simulink model "astrobee"  (R2016b)
settings: configuration reference "cset" (kept outside this file)
PreLoadFcn:
  | astrobee_init;
  | astrobee_prep;
values from neighbouring files (symbols this model uses):
  bus_cmc_msg_ic = Simulink.Bus.createMATLABStruct('cmc_msg')    [bus_init.m]
undefined symbols (not defined in the file or in its folder): ase_local_mode_docking, att_ki, att_kp, center_of_mass, inertia_matrix, mass, mlp_loc_mode_cmd_list, mlp_loc_mode_cmd_times, omega_kd, pos_ki, pos_kp, tun_default_att_ki, tun_default_att_kp, tun_default_center_of_mass, tun_default_inertia_matrix, tun_default_mass, tun_default_omega_kd, tun_default_pos_ki, tun_default_pos_kp, tun_default_vel_kd, vel_kd
libraries: simulink x1, cmc_command_and_mode_control x1, fsw_lib x1, sim_model_lib x1
settings Model: Creator=mjmcinty  LastModifiedBy=jfusco1
settings ConfigSetRef: SourceLocation=Base Workspace

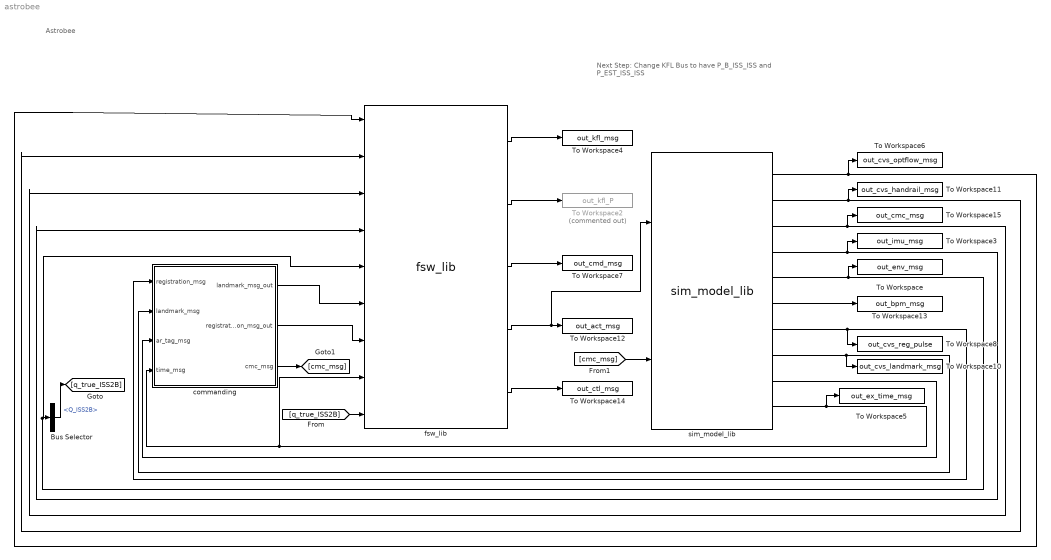
== system astrobee ==
  note: Next Step:
      | Change KFL Bus to have P_B_ISS_ISS and P_EST_ISS_ISS
  note: Astrobee
  Bus Selector : BusSelector  OutputSignals=Q_ISS2B
  To Workspace : ToWorkspace  VariableName=out_env_msg  SaveFormat=Timeseries  SampleTime=-1
  To Workspace10 : ToWorkspace  VariableName=out_cvs_landmark_msg  SaveFormat=Timeseries  SampleTime=-1
  To Workspace11 : ToWorkspace  VariableName=out_cvs_handrail_msg  SaveFormat=Timeseries  SampleTime=-1
  To Workspace12 : ToWorkspace  VariableName=out_act_msg  SaveFormat=Timeseries  SampleTime=-1
  To Workspace13 : ToWorkspace  VariableName=out_bpm_msg  SaveFormat=Timeseries  SampleTime=-1
  To Workspace14 : ToWorkspace  VariableName=out_ctl_msg  SaveFormat=Timeseries  SampleTime=-1
  To Workspace15 : ToWorkspace  VariableName=out_cmc_msg  SaveFormat=Timeseries  SampleTime=-1
  To Workspace2 : ToWorkspace  Commented=on  VariableName=out_kfl_P  SaveFormat=Timeseries  SampleTime=-1
  To Workspace3 : ToWorkspace  VariableName=out_imu_msg  SaveFormat=Timeseries  SampleTime=-1
  To Workspace4 : ToWorkspace  VariableName=out_kfl_msg  SaveFormat=Timeseries  SampleTime=-1
  To Workspace5 : ToWorkspace  VariableName=out_ex_time_msg  SaveFormat=Timeseries  SampleTime=-1
  To Workspace6 : ToWorkspace  VariableName=out_cvs_optflow_msg  SaveFormat=Timeseries  SampleTime=-1
  To Workspace7 : ToWorkspace  VariableName=out_cmd_msg  SaveFormat=Timeseries  SampleTime=-1
  To Workspace8 : ToWorkspace  VariableName=out_cvs_reg_pulse  SaveFormat=Timeseries  SampleTime=-1
  commanding : Subsystem
  fsw_lib : fsw_lib/fsw_lib
  sim_model_lib : sim_model_lib/sim_model_lib
  wires:
  fsw_lib/1 -> To Workspace4/1
  fsw_lib/3 -> To Workspace7/1
  sim_model_lib/5 -> To Workspace/1, fsw_lib/5, Bus Selector/1
  sim_model_lib/4 -> To Workspace3/1, fsw_lib/4
  sim_model_lib/3 -> To Workspace15/1, fsw_lib/3
  sim_model_lib/2 -> To Workspace11/1, fsw_lib/2
  sim_model_lib/1 -> To Workspace6/1, fsw_lib/1
  fsw_lib/2 -> To Workspace2/1
  fsw_lib/4 -> sim_model_lib/1, To Workspace12/1
  fsw_lib/5 -> To Workspace14/1
  sim_model_lib/9 -> commanding/3(ar_tag_msg)
  sim_model_lib/7 -> To Workspace8/1, commanding/1(registration_msg)
  sim_model_lib/10 -> To Workspace5/1, fsw_lib/8, commanding/4(time_msg)
  commanding/1(landmark_msg_out) -> fsw_lib/6
  commanding/2(registration_msg_out) -> fsw_lib/7
  sim_model_lib/8 -> To Workspace10/1, commanding/2(landmark_msg)
  sim_model_lib/6 -> To Workspace13/1
  Bus Selector/1 -> [q_true_ISS2B]  "<Q_ISS2B>"
  commanding/3(cmc_msg) -> [cmc_msg]
  [cmc_msg] -> sim_model_lib/2
  [q_true_ISS2B] -> fsw_lib/9

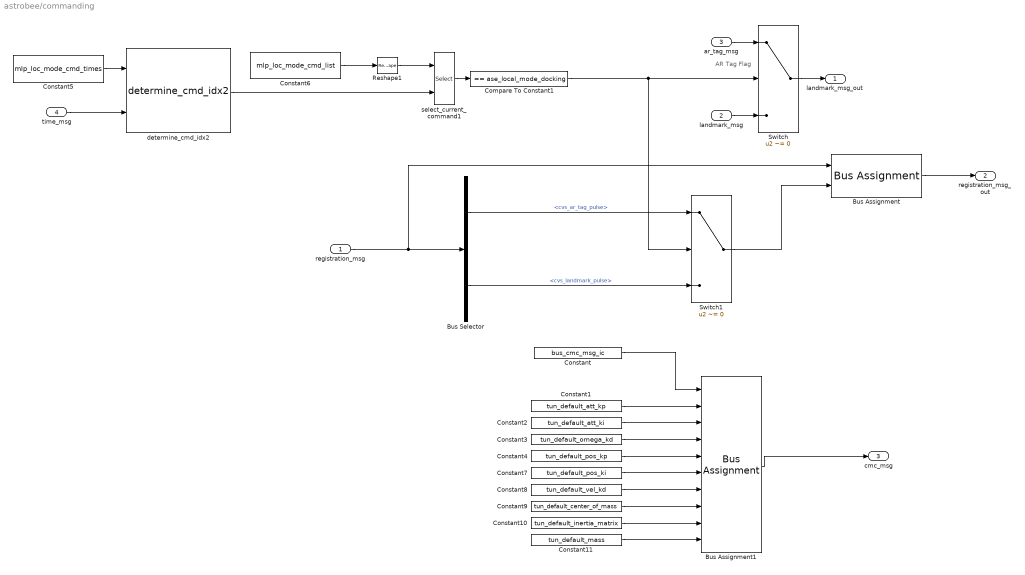
== system astrobee/commanding ==
  note: AR Tag Flag
  registration_msg : Inport  OutDataTypeStr=Bus: cvs_registration_pulse
  landmark_msg : Inport  Port=2
  ar_tag_msg : Inport  Port=3
  time_msg : Inport  Port=4
  Bus Assignment : BusAssignment  AssignedSignals=cvs_landmark_pulse
  Bus Assignment1 : BusAssignment  AssignedSignals=att_kp,att_ki,omega_kd,pos_kp,pos_ki,vel_kd,center_of_mass,inertia_matrix,mass
  Bus Selector : BusSelector  OutputSignals=cvs_ar_tag_pulse,cvs_landmark_pulse
  Compare To Constant1 : simulink/Logic and Bit Operations/Compare To Constant  relop===  const=ase_local_mode_docking  OutDataTypeStr=boolean
  Constant : Constant  Value=bus_cmc_msg_ic  OutDataTypeStr=Bus: cmc_msg
  Constant1 : Constant  Value=tun_default_att_kp
  Constant10 : Constant  Value=tun_default_inertia_matrix
  Constant11 : Constant  Value=tun_default_mass
  Constant2 : Constant  Value=tun_default_att_ki
  Constant3 : Constant  Value=tun_default_omega_kd
  Constant4 : Constant  Value=tun_default_pos_kp
  Constant5 : Constant  Value=mlp_loc_mode_cmd_times
  Constant6 : Constant  Value=mlp_loc_mode_cmd_list
  Constant7 : Constant  Value=tun_default_pos_ki
  Constant8 : Constant  Value=tun_default_vel_kd
  Constant9 : Constant  Value=tun_default_center_of_mass
  Reshape1 : Reshape  OutputDimensionality=Column vector (2-D)
  Switch : Switch  Criteria=u2 ~= 0
  Switch1 : Switch  Criteria=u2 ~= 0
  determine_cmd_idx2 : cmc_command_and_mode_control/cmc_command_and_mode_control/determine_cmd_idx2
  select_current_command1 : Selector  NumberOfDimensions=2  InputPortWidth=3  IndexOptions=Index vector (port),Select all  Indices=[1 3],1  OutputSizes=1,1
  landmark_msg_out : Outport
  registration_msg_out : Outport  Port=2
  cmc_msg : Outport  Port=3  OutDataTypeStr=Bus: cmc_msg
  wires:
  time_msg/1 -> determine_cmd_idx2/2
  select_current_command1/1 -> Compare To Constant1/1
  Constant5/1 -> determine_cmd_idx2/1
  determine_cmd_idx2/1 -> select_current_command1/2
  Constant6/1 -> Reshape1/1
  Reshape1/1 -> select_current_command1/1
  ar_tag_msg/1 -> Switch/1
  landmark_msg/1 -> Switch/3
  Switch/1 -> landmark_msg_out/1
  Compare To Constant1/1 -> Switch1/2, Switch/2
  registration_msg/1 -> Bus Assignment/1, Bus Selector/1
  Bus Selector/1 -> Switch1/1  "<cvs_ar_tag_pulse>"
  Bus Selector/2 -> Switch1/3  "<cvs_landmark_pulse>"
  Bus Assignment/1 -> registration_msg_out/1
  Switch1/1 -> Bus Assignment/2
  Bus Assignment1/1 -> cmc_msg/1
  Constant/1 -> Bus Assignment1/1
  Constant3/1 -> Bus Assignment1/4
  Constant4/1 -> Bus Assignment1/5
  Constant2/1 -> Bus Assignment1/3
  Constant7/1 -> Bus Assignment1/6
  Constant1/1 -> Bus Assignment1/2
  Constant8/1 -> Bus Assignment1/7
  Constant9/1 -> Bus Assignment1/8
  Constant10/1 -> Bus Assignment1/9
  Constant11/1 -> Bus Assignment1/10
